simulink model "EstimationSimulations"  (R2024b)
settings: Solver=VariableStepAuto  StartTime=0.0  StopTime=300  RelTol=1e-3
undefined symbols (not defined in the file): bias, k1, k2, r_noise, use_noise, yaw_0, yaw_noise
libraries: simulink x2
settings Model: Creator=ricar  LastModifiedBy=ricar

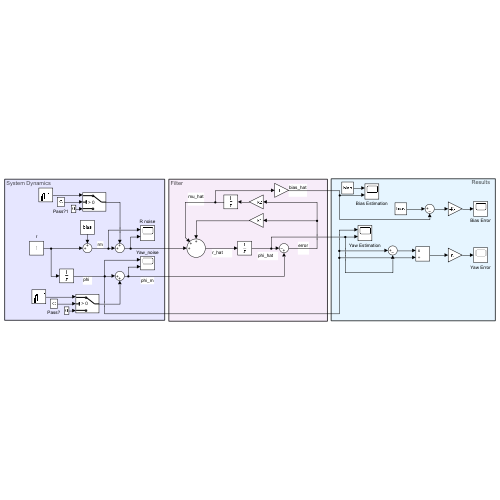
[thumbnail: Simulink's stored preview of the top-level diagram]
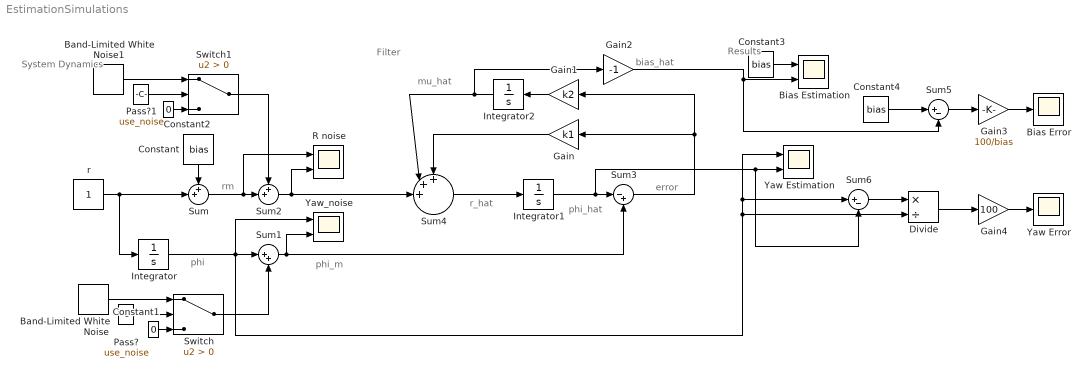
== system EstimationSimulations ==
  note: Results
  note: mu_hat
  note: Filter
  note: error
  note: phi_hat
  note: System Dynamics
  note: rm
  note: phi
  note: r_hat
  note: phi_m
  note: bias_hat
  Band-Limited White Noise : simulink/Sources/Band-Limited White Noise  Cov=[yaw_noise]  Ts=0.1  seed=[10576]
  Band-Limited White Noise1 : simulink/Sources/Band-Limited White Noise  Cov=[r_noise]  Ts=0.1  seed=[1]
  Bias Error : Scope
  Bias Estimation : Scope  NumInputPorts=2
  Constant : Constant  Value=bias
  Constant1 : Constant  Value=0
  Constant2 : Constant  Value=0
  Constant3 : Constant  Value=bias
  Constant4 : Constant  Value=bias
  Divide : Product  Inputs=*/
  Gain : Gain  Gain=k1
  Gain1 : Gain  Gain=k2
  Gain2 : Gain  Gain=-1
  Gain3 : Gain  Gain=100/bias
  Gain4 : Gain  Gain=100
  Integrator : Integrator  InitialCondition=yaw_0
  Integrator1 : Integrator
  Integrator2 : Integrator
  Pass? : Constant  Value=use_noise
  Pass?1 : Constant  Value=use_noise
  R noise : Scope  NumInputPorts=2
  Sum : Sum  Inputs=++|
  Sum1 : Sum  Inputs=|++
  Sum2 : Sum  Inputs=++|
  Sum3 : Sum  Inputs=|-+
  Sum4 : Sum  Inputs=+++||
  Sum5 : Sum  Inputs=|+-
  Sum6 : Sum  Inputs=|+-
  Switch : Switch  Criteria=u2 > Threshold  SaturateOnIntegerOverflow=off  InputSameDT=off
  Switch1 : Switch  Criteria=u2 > Threshold  SaturateOnIntegerOverflow=off  InputSameDT=off
  Yaw Error : Scope
  Yaw Estimation : Scope  NumInputPorts=2
  Yaw_noise : Scope  NumInputPorts=2
  r : Constant
  wires:
  r/1 -> Integrator/1, Sum/2
  Constant/1 -> Sum/1
  Integrator/1 -> Divide/2, Yaw Estimation/1, Sum6/1, Yaw_noise/1, Sum1/1
  Sum1/1 -> Yaw_noise/2, Sum3/2
  Pass?/1 -> Switch/2
  Constant1/1 -> Switch/3
  Band-Limited White Noise/1 -> Switch/1
  Switch/1 -> Sum1/2
  Sum/1 -> R noise/1, Sum2/2
  Constant2/1 -> Switch1/3
  Pass?1/1 -> Switch1/2
  Band-Limited White Noise1/1 -> Switch1/1
  Switch1/1 -> Sum2/1
  Sum2/1 -> R noise/2, Sum4/3
  Integrator1/1 -> Sum6/2, Yaw Estimation/2, Sum3/1
  Sum4/1 -> Integrator1/1
  Gain/1 -> Sum4/1
  Sum3/1 -> Gain1/1, Gain/1
  Gain1/1 -> Integrator2/1
  Integrator2/1 -> Gain2/1, Sum4/2
  Constant3/1 -> Bias Estimation/1
  Gain2/1 -> Bias Estimation/2, Sum5/2
  Constant4/1 -> Sum5/1
  Sum5/1 -> Gain3/1
  Gain3/1 -> Bias Error/1
  Sum6/1 -> Divide/1
  Divide/1 -> Gain4/1
  Gain4/1 -> Yaw Error/1
